simulink model "personal_transporter_model2_with_nonidealities"  (R2017a)
settings: Solver=VariableStepAuto  StartTime=0.0  StopTime=final_time  FixedStep=Ts  MaxStep=1  RelTol=1e-2
values from neighbouring files (symbols this model uses):
  alpha_c = 0.999    [digital_filters.m]
  beta_c = 1-alpha_c    (= 0.001)    [digital_filters.m]
  C_2 = [c11_2    0       -c11_2    0;      0      c11_2     -c11_2    0;      -c11_2   -c11_2    c33_2     c34_2;      0      0       c34_2     -c34_2]    [overall_model_2.m]
  D = 0.4    [param_personal_transporter_2_backup.m]    (also in vehicle_params.m = 0.5)
  Dec_2 = inv([1 1 0;0 0 1; 1 -1 0])    [overall_model_2.m]
  g = 9.81    [param_personal_transporter_2_backup.m]    (also in vehicle_params.m)
  iMAX = 2*iNom    (= 40)    [vehicle_params.m]
  k_PLL = 15    [digital_filters.m]
  k_s = 1440    [param_personal_transporter_2_backup.m]    (also in vehicle_params.m = 850)
  K_steer = dlqr(A_td,B_td,Q_steer,R_steer)    [steering_model_and_controller.m]
  Kd = dlqr(Ad,Bd,Q,R)    [equilibrium_model_and_controller.m]
  kt = ke    (= 0.0353677651315)    [param_personal_transporter_2_backup.m]    (also in vehicle_params.m = 0.694)
  L = P*C'*inv(C*P*C'+R)    [f_updating.m]    (also in f_updating_e.m; param_personal_transporter_2_backup.m = 0.9; vehicle_params.m = 0.1)
  m_P = 80    [param_personal_transporter_2_backup.m]    (also in vehicle_params.m = 30)
  n_hall = 3    [vehicle_params.m]
  r = 0.1    [param_personal_transporter_2_backup.m]    (also in vehicle_params.m)
  R_kalman_IMU = 20    [digital_filters.m]
  references_dot_delta = [  0 ,0;                         20, 0;                         23, 1;                         26, -1;                         29, 0;                         final_time, 0]    [steering_model_and_controller.m]
  references_dot_Xb = [ 0, 0;                     2.5, 0.5;                     5, 0;                     final_time, 0]    [equilibrium_model_and_controller.m]
  S = [ r/2  r/2  0;       r/D  -r/D 0;       0     0   1]    [overall_model.m]    (also in param_personal_transporter_2_backup.m = [ r/2  r/2  0  0;       r/D  -r/D 0  0;       0     0   1  0)
  S_2 = [ r/2  r/2  0  0;       r/D  -r/D 0  0;       0     0   1  0;       0     0   0  1]    [overall_model_2.m]
  Smot = [ rho  0   1;        0   rho  1;        0    0   1]    [overall_model.m]
  tacho_to_angle = (2*pi)/(n_poles*n_hall)    [vehicle_params.m]
  tau_PLL = omega_PLL    (= 31.4159265359)    [digital_filters.m]
  Ts = 0.01    [angle_fusion_readings.m]    (also in imu_model.m; other_stuff.m; param_personal_transporter.m; param_personal_transporter_2.m)
  U_2 = [1/rho 0 0;0 1/rho 0; -1/rho -1/rho -1; 0 0 1]    [overall_model_2.m]
undefined symbols (not defined in the file or in its folder): denF, denIloop, denIMU, denIMUint, denPI, denTorques, Discrete, n_poles, numF, numIloop, numIMU, numIMUint, numPI, numTorques, Time
libraries: simulink x5, ctrlSharedLib x2, cstblocks x1
settings Model: Creator=Dino Spiller  LastModifiedBy=mac_daino
settings SolverCC: ZeroCrossControl=DisableAll  InsertRTBMode=Never (minimum delay)
settings DataIOCC: LimitDataPoints=on  SaveFormat=Array  SignalLoggingSaveFormat=ModelDataLogs
settings OptimizationCC: ExpressionDepthLimit=2147483647  LifeSpan=inf
settings DebuggingCC: UnderspecifiedInitializationDetection=Classic  MergeDetectMultiDrivingBlocksExec=none  SolverPrmCheckMsg=warning  FcnCallInpInsideContextMsg=warning  StateNameClashWarn=warning  SFUnexpectedBacktrackingDiag=warning  SFNoUnconditionalDefaultTransitionDiag=warning  SFExecutionAtInitializationDiag=none
settings HardwareCC: ProdBitPerPointer=32  ProdBitPerSizeT=32  ProdBitPerPtrDiffT=32  ProdLargestAtomicFloat=None  ProdIntDivRoundTo=Undefined  ProdEndianess=Unspecified  ProdWordSize=32  ProdHWDeviceType=32-bit Generic
settings ModelReferenceCC: ModelReferenceMinAlgLoopOccurrences=on  PropagateSignalLabelsOutOfModel=off
settings RTWCC: CheckMdlBeforeBuild=Warning
settings GRTTargetCC: TargetLangStandard=C89/C90 (ANSI)  GeneratePreprocessorConditionals=Disable all  CombineOutputUpdateFcns=off  GRTInterface=on
settings ConfigComp: CovMetricSettings=dw  CovHtmlReporting=on  CovSaveCumulativeToWorkspaceVar=on  CovSaveSingleToWorkspaceVar=on  CovExternalEMLEnable=off

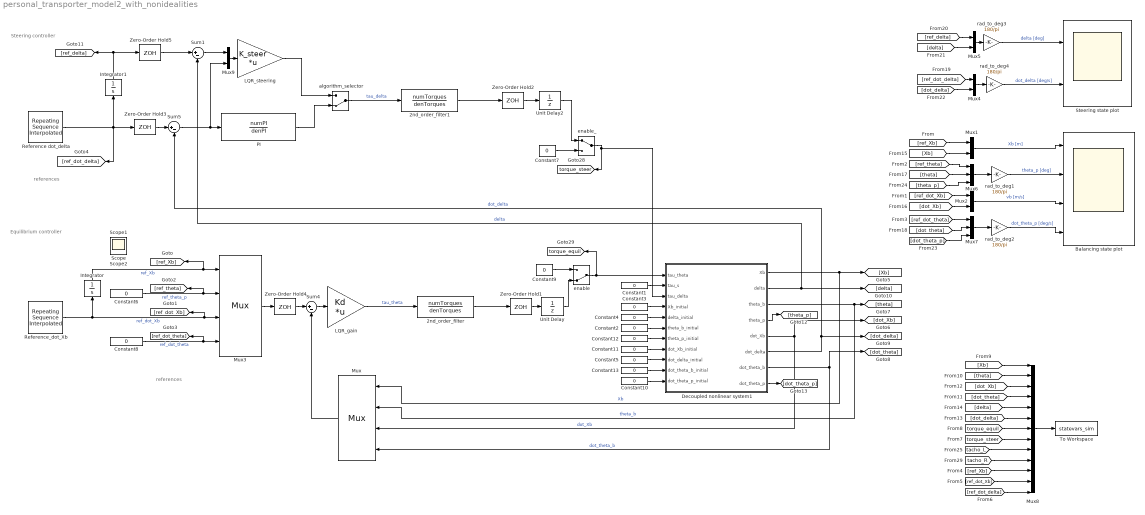
== system personal_transporter_model2_with_nonidealities ==
  note: Steering controller
  note: references
  note: Equilibrium controller
  note: references
  2nd_order_filter : DiscreteTransferFcn  Numerator=numTorques  Denominator=denTorques
  2nd_order_filter1 : DiscreteTransferFcn  Numerator=numTorques  Denominator=denTorques
  Balancing state plot : Scope  NumInputPorts=4
  Constant{1..13} (13 alike) : Constant  Value=0
  Decoupled nonlinear system1 : Subsystem
  Integrator : Integrator
  Integrator1 : Integrator
  LQR_gain : Gain  Gain=Kd  Multiplication=Matrix(K*u)
  LQR_steering : Gain  Gain=K_steer  Multiplication=Matrix(K*u)
  Mux : Mux
      settings: DisplayOption=signals
  Mux{1..2,4..5,9} (5 alike) : Mux  Inputs=2
  Mux3 : Mux
      settings: DisplayOption=signals
  Mux6 : Mux  Inputs=3
  Mux7 : Mux  Inputs=3
  Mux8 : Mux  Inputs=13
  PI : DiscreteTransferFcn  Numerator=numPI  Denominator=denPI
  Reference dot_delta : simulink/Sources/Repeating Sequence Interpolated  OutValues=references_dot_delta(:,2)  TimeValues=references_dot_delta(:,1)  LookUpMeth=Interpolation-Use End Values  tsamp=Ts  OutMin=[]  OutMax=[]  OutDataTypeStr=double  OutputDataTypeScalingMode=double  OutDataType=fixdt(0,8)  OutScaling=2^-10
  Reference_dot_Xb : simulink/Sources/Repeating Sequence Interpolated  OutValues=references_dot_Xb(:,2)  TimeValues=references_dot_Xb(:,1)  LookUpMeth=Interpolation-Use End Values  tsamp=Ts  OutMin=[]  OutMax=[]  OutDataTypeStr=double  OutputDataTypeScalingMode=double  OutDataType=fixdt(0,8)  OutScaling=2^-10
  Steering state plot : Scope  NumInputPorts=2
  Sum1 : Sum  Inputs=|+-
  Sum4 : Sum  Inputs=|+-
  Sum5 : Sum  Inputs=|+-
  To Workspace : ToWorkspace  VariableName=statevars_sim  SaveFormat=Timeseries  SampleTime=Ts
  Unit Delay : UnitDelay  SampleTime=Ts
  Unit Delay2 : UnitDelay  SampleTime=Ts
  Zero-Order Hold{1..5} (5 alike) : ZeroOrderHold  SampleTime=Ts
  algorithm_selector : ManualSwitch  CurrentSetting=0
  enable : ManualSwitch  CurrentSetting=0
  enable_ : ManualSwitch
  rad_to_deg{1..4} (4 alike) : Gain  Gain=180/pi
  Scope : Scope
  Scope1 : Scope
  Scope2 : Scope
  tag scope: torque_equil=global, torque_steer=global
  wires:
  Reference_dot_Xb/1 -> [ref_dot_Xb], Mux3/3, Integrator/1  "ref_dot_Xb"
  Decoupled nonlinear system1/1(Xb) -> [Xb], Mux/1  "Xb"
  Decoupled nonlinear system1/3(theta_b) -> [theta], Mux/2  "theta_b"
  Decoupled nonlinear system1/2(delta) -> Sum1/2, [delta]  "delta"
  Decoupled nonlinear system1/6(dot_delta) -> Sum5/2, [dot_delta]  "dot_delta"
  Constant3/1 -> Decoupled nonlinear system1/4(Xb_initial)
  Constant4/1 -> Decoupled nonlinear system1/5(delta_initial)
  Constant11/1 -> Decoupled nonlinear system1/8(dot_Xb_initial)
  Constant5/1 -> Decoupled nonlinear system1/9(dot_delta_initial)
  Constant10/1 -> Decoupled nonlinear system1/11(dot_theta_p_initial)
  enable/1 -> [torque_equil], Decoupled nonlinear system1/1("tau_theta ")
  Constant6/1 -> [ref_theta], Mux3/2  "ref_theta_p"
  Reference dot_delta/1 -> [ref_dot_delta], Zero-Order Hold3/1, Integrator1/1
  Constant7/1 -> enable_/2
  Zero-Order Hold2/1 -> Unit Delay2/1
  Mux4/1 -> rad_to_deg4/1
  Mux5/1 -> rad_to_deg3/1
  Integrator/1 -> [ref_Xb], Mux3/1  "ref_Xb"
  Constant8/1 -> [ref_dot_theta], Mux3/4  "ref_dot_theta"
  Mux3/1 -> Zero-Order Hold4/1
  Sum4/1 -> LQR_gain/1
  Mux/1 -> Sum4/2
  Sum5/1 -> Mux9/2, PI/1
  Mux1/1 -> Balancing state plot/1  "Xb [m]"
  [ref_Xb] -> Mux1/1
  [ref_dot_Xb] -> Mux2/1
  Zero-Order Hold4/1 -> Sum4/1
  Zero-Order Hold1/1 -> Unit Delay/1
  Mux8/1 -> To Workspace/1
  [torque_steer] -> Mux8/8
  [torque_equil] -> Mux8/7
  [tacho_L] -> Mux8/9
  [tacho_R] -> Mux8/10
  [ref_Xb] -> Mux8/11
  [ref_dot_Xb] -> Mux8/12
  [ref_dot_delta] -> Mux8/13
  Constant9/1 -> enable/1
  Unit Delay/1 -> enable/2
  [Xb] -> Mux8/1
  [theta] -> Mux8/2
  [dot_Xb] -> Mux8/3
  [dot_theta] -> Mux8/4
  [dot_delta] -> Mux8/6
  [delta] -> Mux8/5
  [Xb] -> Mux1/2
  [dot_Xb] -> Mux2/2
  Mux6/1 -> rad_to_deg1/1
  Mux2/1 -> Balancing state plot/3  "vb [m/s]"
  rad_to_deg1/1 -> Balancing state plot/2  "theta_p [deg]"
  [ref_theta] -> Mux6/1
  [theta] -> Mux6/2
  [ref_dot_theta] -> Mux7/1
  [dot_theta] -> Mux7/2
  Mux7/1 -> rad_to_deg2/1
  rad_to_deg2/1 -> Balancing state plot/4  "dot_theta_p [deg/s]"
  Unit Delay2/1 -> enable_/1
  Integrator1/1 -> Zero-Order Hold5/1, [ref_delta]
  rad_to_deg3/1 -> Steering state plot/1  "delta [deg]"
  rad_to_deg4/1 -> Steering state plot/2  "dot_delta [deg/s]"
  Zero-Order Hold3/1 -> Sum5/1
  Sum1/1 -> Mux9/1
  Mux9/1 -> LQR_steering/1
  LQR_steering/1 -> algorithm_selector/1
  PI/1 -> algorithm_selector/2
  algorithm_selector/1 -> 2nd_order_filter1/1  "tau_delta"
  [dot_delta] -> Mux4/2
  [ref_dot_delta] -> Mux4/1
  [delta] -> Mux5/2
  [ref_delta] -> Mux5/1
  Zero-Order Hold5/1 -> Sum1/1
  LQR_gain/1 -> 2nd_order_filter/1  "tau_theta"
  2nd_order_filter/1 -> Zero-Order Hold1/1
  enable_/1 -> Decoupled nonlinear system1/3(tau_delta), [torque_steer]
  2nd_order_filter1/1 -> Zero-Order Hold2/1
  Constant1/1 -> Decoupled nonlinear system1/2(tau_s)
  Constant2/1 -> Decoupled nonlinear system1/6(theta_b_initial)
  Constant12/1 -> Decoupled nonlinear system1/7(theta_p_initial)
  Constant13/1 -> Decoupled nonlinear system1/10(dot_theta_b_initial)
  Decoupled nonlinear system1/5("dot_Xb ") -> Mux/3, [dot_Xb]  "dot_Xb"
  Decoupled nonlinear system1/7(dot_theta_b) -> Mux/4, [dot_theta]  "dot_theta_b"
  Decoupled nonlinear system1/4(theta_p) -> [theta_p]
  Decoupled nonlinear system1/8(dot_theta_p) -> [dot_theta_p]
  [theta_p] -> Mux6/3
  [dot_theta_p] -> Mux7/3

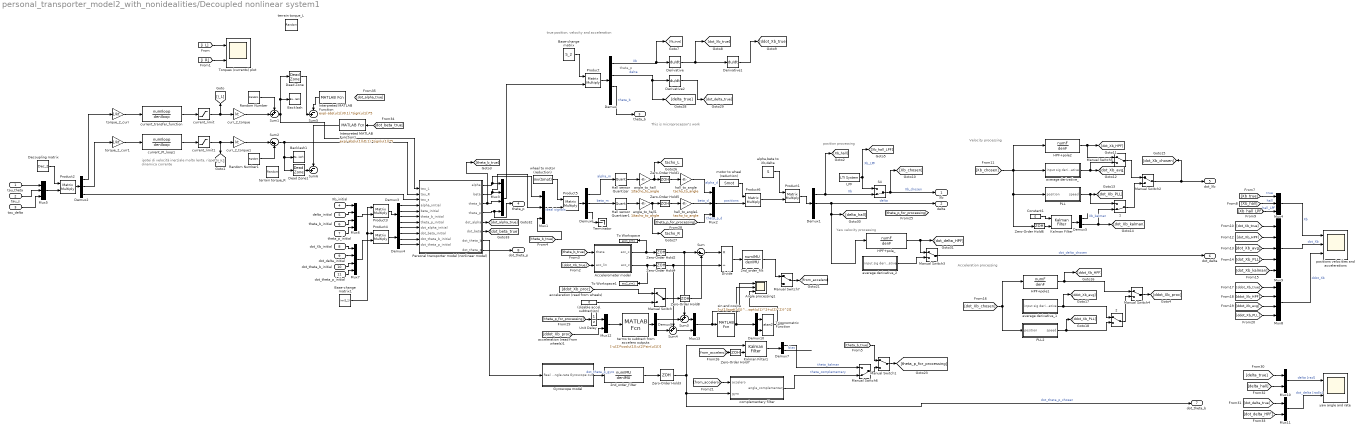
== system personal_transporter_model2_with_nonidealities/Decoupled nonlinear system1 ==
  note: theta_p
  note: ipotei di velocità  inerziale molto lenta, rispetto
      | a dinamica corrente
  note: Velocity processing
  note: Acceleration processing
  note: true position, velocity and acceleration
  note: position processing
  note: Yaw velocity processing
  note: This is microprocessor's work
  "tau_theta " : Inport
  tau_s : Inport  Port=2
  tau_delta : Inport  Port=3
  Xb_initial : Inport  Port=4
  delta_initial : Inport  Port=5
  theta_b_initial : Inport  Port=6
  theta_p_initial : Inport  Port=7
  dot_Xb_initial : Inport  Port=8
  dot_delta_initial : Inport  Port=9
  dot_theta_b_initial : Inport  Port=10
  dot_theta_p_initial : Inport  Port=11
  (disable accel. subtraction) : Constant  Value=0
  1 : ManualSwitch  CurrentSetting=0
  2 : ManualSwitch
  2nd_order_filt : DiscreteTransferFcn  Numerator=numIMU  Denominator=denIMU
  2nd_order_filter : DiscreteTransferFcn  Numerator=numIMU  Denominator=denIMU
  Accelerometer model : Subsystem
  Angle processing1 : Scope  NumInputPorts=3
  Backlash : Backlash  BacklashWidth=1.8
  Backlash1 : Backlash
  Base-change matrix : Constant  Value=S_2  VectorParams1D=off
  Base-change matrix1 : Constant  Value=inv(S_2)  VectorParams1D=off
  Constant1 : Constant  Value=0
  Dead Zone : DeadZone  LowerValue=-2  UpperValue=2  SaturateOnIntegerOverflow=on
  Dead Zone1 : DeadZone  LowerValue=-2  UpperValue=2  SaturateOnIntegerOverflow=on
  Decoupling matrix : Constant  Value=Dec_2  VectorParams1D=off
  Demux : Demux
  Demux1 : Demux  Outputs=3
  Demux{5,7,9..10} (4 alike) : Demux  Outputs=2
  Demux2 : Demux  Outputs=3
  Demux3 : Demux
  Demux4 : Demux
  Demux6 : Demux  Outputs=3
  Derivative : Derivative
  Derivative1 : Derivative
  Derivative2 : Derivative
  Divide : Product  Inputs=*/
  Gyroscope model : Subsystem
  HPF+pole1 : DiscreteTransferFcn  Numerator=numF  Denominator=denF  SampleTime=Ts
  HPF+pole2 : DiscreteTransferFcn  Numerator=numF  Denominator=denF  SampleTime=Ts
  HPF+pole_ : DiscreteTransferFcn  Numerator=numF  Denominator=denF
  Hall sensor Quantizer : Quantizer  QuantizationInterval=(2*pi)/(n_poles*n_hall)
  Hall sensor Quantizer1 : Quantizer  QuantizationInterval=(2*pi)/(n_poles*n_hall)
  Interpreted MATLAB Function : MATLABFcn  MATLABFcn=exp(-abs(u(1))/0.1).*sign(u(1))*5  OutputDimensions=[1]
  Interpreted MATLAB Function1 : MATLABFcn  MATLABFcn=exp(-abs(u(1))/0.1).*sign(u(1))*5  OutputDimensions=[1]
  Kalman Filter : ctrlSharedLib/Kalman Filter  TimeDomain=Discrete-Time  UseCurrentEstimator=on  ModelSource=Individual A, B, C, D matrices  ModelSourceVariable=ss(0.95,1,1,0,1)  A=[1 Ts; 0 1]  B=[0 ; 0]  C=[1 0]  D=0  NumberOfStates=1  NumberOfInputs=1  NumberOfOutputs=1  InitialEstimateSource=Dialog  X0=0  P0=10  UseK=off  UseGH=off  NumberOfProcessNoiseInputs=1  G=1  TimeInvariantG=on  H=0  TimeInvariantH=on  Q=[ 0.0001 0; 0 0.1]  TimeInvariantQ=on  R=4.06e-3  TimeInvariantR=on  N=0  TimeInvariantN=on  AddInputPort=on  AddEnablePort=off  OutputEstimatedY=off  OutputP=off  Ts=-1
  Kalman Filter1 : ctrlSharedLib/Kalman Filter  TimeDomain=Discrete-Time  UseCurrentEstimator=on  ModelSource=Individual A, B, C, D matrices  ModelSourceVariable=ss(0.95,1,1,0,1)  A=[1 -Ts; 0 1]  B=[Ts ; 0]  C=[1 0]  D=0  NumberOfStates=1  NumberOfInputs=1  NumberOfOutputs=1  InitialEstimateSource=Dialog  X0=0  P0=10  UseK=off  UseGH=off  NumberOfProcessNoiseInputs=1  G=1  TimeInvariantG=on  H=0  TimeInvariantH=on  Q=Q_kalman_IMU  TimeInvariantQ=on  R=R_kalman_IMU  TimeInvariantR=on  N=0  TimeInvariantN=on  AddInputPort=on  AddEnablePort=off  OutputEstimatedY=off  OutputP=off  Ts=-1
  LPF : cstblocks/LTI System  sys=LPF_c  IC=[]
  Manual Switch{,1..5,7} (7 alike) : ManualSwitch
  Manual Switch6 : ManualSwitch  CurrentSetting=0
  Mux{1..2,4..5} (4 alike) : Mux  Inputs=3
  Mux{10..13} (4 alike) : Mux  Inputs=2
  Mux{3,6..8} (4 alike) : Mux
  Mux9 : Mux  Inputs=5
  PLL : Subsystem
  PLL2 : Subsystem
  Personal transporter model (nonlinear model) : Subsystem
  Product{,1..6} (7 alike) : Product  Multiplication=Matrix(*)  RndMeth=Zero
  Random Number : RandomNumber  Variance=0.1  SampleTime=Ts
  Random Number1 : RandomNumber  Variance=0.1  Seed=50  SampleTime=Ts
  S4 : ManualSwitch  CurrentSetting=0
  Sum : Sum  Inputs=|+-
  Sum1 : Sum  Inputs=++|
  Sum2 : Sum  Inputs=|++
  Sum3 : Sum  Inputs=++|
  Sum4 : Sum  Inputs=++|
  Sum5 : Sum  Inputs=-+|
  Sum6 : Sum  Inputs=-+|
  Terminator : Terminator
  To Workspace : ToWorkspace  VariableName=accX_sim1  SaveFormat=Timeseries  SampleTime=-1
  To Workspace1 : ToWorkspace  VariableName=accZ_sim1  SaveFormat=Timeseries  SampleTime=-1
  Torques (currents) plot : Scope  NumInputPorts=2
  Trigonometric Function : Trigonometry  Operator=atan2
  Unit Delay : UnitDelay  InitialCondition=0.001  SampleTime=-1
  Zero-Order Hold{1..8} (8 alike) : ZeroOrderHold  SampleTime=Ts
  alpha,beta to Xb,delta : Constant  Value=S  VectorParams1D=off
  angle_to_hall : Gain  Gain=1/tacho_to_angle
  angle_to_hall1 : Gain  Gain=1/tacho_to_angle
  average derivative_ : Subsystem
  average derivative_1 : Subsystem
  average derivative_2 : Subsystem
  complementary filter : Subsystem
  curr_2_torque : Gain  Gain=kt
  curr_2_torque1 : Gain  Gain=kt
  current_PI_loop1 : DiscreteTransferFcn  Numerator=numIloop  Denominator=denIloop
  current_limit : Saturate  UpperLimit=iMAX  LowerLimit=-iMAX  LinearizeAsGain=off
  current_limit1 : Saturate  UpperLimit=iMAX  LowerLimit=-iMAX  LinearizeAsGain=off
  current_transfer_function : DiscreteTransferFcn  Numerator=numIloop  Denominator=denIloop
  hall_to_angle : Gain  Gain=tacho_to_angle
  hall_to_angle1 : Gain  Gain=tacho_to_angle
  motor to wheel (reduction) : Constant  Value=Smot  VectorParams1D=off
  positions velocities and accelerations : Scope  NumInputPorts=3
  sin and cosine : MATLABFcn  MATLABFcn=[-u(1)/sqrt(u(1)^2+u(2)^2); sqrt(1-(u(1)/sqrt(u(1)^2+u(2)^2))^2)]  OutputDimensions=[2,1]  Output1D=off
  terms to subtract from accelero outputs : MATLABFcn  MATLABFcn=[-u(2)*cos(u(1));u(2)*sin(u(1))]  OutputDimensions=[2,1]  Output1D=off
  terrain torque_L : UniformRandomNumber  Minimum=-0.1  Maximum=0.1  SampleTime=Ts
  terrain torque_R : UniformRandomNumber  Minimum=-0.1  Maximum=0.1  Seed=100  SampleTime=Ts
  torque_2_curr : Gain  Gain=1/kt
  torque_2_curr1 : Gain  Gain=1/kt
  wheel to motor (reduction) : Constant  Value=inv(Smot)  VectorParams1D=off
  yaw angle and rate : Scope  NumInputPorts=2
  Xb : Outport
  delta : Outport  Port=2
  theta_b : Outport  Port=3
  theta_p : Outport  Port=4
  "dot_Xb " : Outport  Port=5
  dot_delta : Outport  Port=6
  dot_theta_b : Outport  Port=7
  dot_theta_p : Outport  Port=8
  tag scope: tacho_L=global, tacho_R=global
  wires:
  Base-change matrix1/1 -> Product3/1, Product4/1
  dot_delta_initial/1 -> Mux7/2
  Decoupling matrix/1 -> Product2/1
  Product4/1 -> Demux4/1
  Mux7/1 -> Product4/2
  Demux3/2 -> Personal transporter model (nonlinear model)/5(beta_initial)
  Product3/1 -> Demux3/1
  Demux3/1 -> Personal transporter model (nonlinear model)/4(alpha_initial)
  Mux5/1 -> Product2/2
  Base-change matrix/1 -> Product/1
  Demux4/2 -> Personal transporter model (nonlinear model)/9(dot_beta_initial)
  Xb_initial/1 -> Mux6/1
  Demux4/1 -> Personal transporter model (nonlinear model)/8(dot_alpha_initial)
  delta_initial/1 -> Mux6/2
  dot_Xb_initial/1 -> Mux7/1
  Mux6/1 -> Product3/2
  Mux3/1 -> Product/2
  Demux/1 -> [Xb_true], Derivative/1  "Xb"
  Product/1 -> Demux/1
  Product2/1 -> Demux2/1
  "tau_theta "/1 -> Mux5/1
  Demux/2 -> Derivative2/1, [delta_true]  "delta"
  Personal transporter model (nonlinear model)/3(theta_b) -> [theta_b_true], Mux3/3
  Personal transporter model (nonlinear model)/4(theta_p) -> theta_p/1, Mux3/4
  Demux/3 -> theta_b/1  "theta_b"
  Demux3/4 -> Personal transporter model (nonlinear model)/7(theta_p_initial)
  Demux3/3 -> Personal transporter model (nonlinear model)/6(theta_b_initial)
  Demux4/3 -> Personal transporter model (nonlinear model)/10(dot_theta_b_initial)
  Demux4/4 -> Personal transporter model (nonlinear model)/11(dot_theta_p_initial)
  theta_p_initial/1 -> Mux6/4
  theta_b_initial/1 -> Mux6/3
  dot_theta_b_initial/1 -> Mux7/3
  dot_theta_p_initial/1 -> Mux7/4
  tau_s/1 -> Mux5/2
  tau_delta/1 -> Mux5/3
  Demux2/3 -> Personal transporter model (nonlinear model)/3(tau_s)
  current_limit1/1 -> curr_2_torque1/1, [i_R]
  [i_L] -> Torques (currents) plot/1
  Demux2/1 -> torque_2_curr/1
  curr_2_torque/1 -> Sum1/2
  Demux2/2 -> torque_2_curr1/1
  Sum1/1 -> Personal transporter model (nonlinear model)/1("tau_L "), Dead Zone/1, Backlash/1
  curr_2_torque1/1 -> Sum2/1
  torque_2_curr/1 -> current_transfer_function/1
  [i_R] -> Torques (currents) plot/2
  current_limit/1 -> [i_L], curr_2_torque/1
  Sum2/1 -> Personal transporter model (nonlinear model)/2("tau_R "), Backlash1/1, Dead Zone1/1
  Interpreted MATLAB Function1/1 -> Sum6/1
  [dot_beta_true] -> Interpreted MATLAB Function1/1
  current_PI_loop1/1 -> current_limit1/1
  torque_2_curr1/1 -> current_PI_loop1/1
  Random Number1/1 -> Sum2/2
  Interpreted MATLAB Function/1 -> Sum5/1
  Random Number/1 -> Sum1/1
  Dead Zone1/1 -> Sum6/2
  Dead Zone/1 -> Sum5/2
  current_transfer_function/1 -> current_limit/1
  Demux10/1 -> Trigonometric Function/1
  Zero-Order Hold6/1 -> Kalman Filter/2
  Zero-Order Hold7/1 -> Kalman Filter1/2
  Demux6/2 -> Hall sensor Quantizer1/1  "beta_m"
  Personal transporter model (nonlinear model)/1(alpha) -> Mux1/1, Mux3/1
  Demux6/1 -> Hall sensor Quantizer/1  "alpha_m"
  [ddot_Xb_HPF] -> Mux8/2
  wheel to motor (reduction)/1 -> Product5/1
  [delta_true] -> Mux10/1
  Personal transporter model (nonlinear model)/7(dot_theta_b) -> Gyroscope model/1(Real angle-rate)
  average derivative_/1(derivative) -> [dot_Xb_avg], Manual Switch5/2
  [ddot_Xb_true] -> Accelerometer model/2(acc_lin)
  angle_to_hall1/1 -> Zero-Order Hold5/1, [tacho_R]
  Manual Switch2/1 -> "dot_Xb "/1, [dot_Xb_chosen]
  [delta_hall] -> Mux10/2
  Mux1/1 -> Product5/2  "ideal signals"
  Demux7/2 -> ?  "bias"
  PLL/1("speed ") -> [dot_Xb_PLL], 1/1
  [dot_Xb_avg] -> Mux9/3
  [dot_delta_true] -> Mux11/1
  Accelerometer model/2(acc_z) -> To Workspace1/1, Zero-Order Hold4/1
  sin and cosine/1 -> Demux10/1, Angle processing1/2
  hall_to_angle/1 -> Mux2/1  "alpha_d"
  angle_to_hall/1 -> [tacho_L], Zero-Order Hold1/1
  Product6/1 -> Product1/2
  Manual Switch3/1 -> dot_delta/1  "dot_delta_chosen"
  Mux11/1 -> yaw angle and rate/2  "dot_delta [rad/s]"
  (disable accel. subtraction)/1 -> Manual Switch/2
  Mux2/1 -> Product6/2  "positions"
  LPF/1 -> [Xb_hall_LPF], S4/1  "Xb_LPF"
  Personal transporter model (nonlinear model)/2(beta) -> Mux1/2, Mux3/2
  Manual Switch5/1 -> Manual Switch2/1
  alpha,beta to Xb,delta/1 -> Product1/1
  Manual Switch1/1 -> [theta_p_for_processing]
  Constant1/1 -> Kalman Filter/1
  [Xb_hall_LPF] -> Mux4/3  "hall_LPF"
  Demux1/2 -> delta/1, [delta_hall], HPF+pole_/1  "delta"
  Derivative1/1 -> [ddot_Xb_true]
  [dot_Xb_kalman] -> Mux9/5
  HPF+pole1/1 -> [ddot_Xb_HPF], Manual Switch4/1
  [theta_b_true] -> Accelerometer model/1(theta)
  Mux4/1 -> positions velocities and accelerations/1  "Xb"
  [dot_Xb_HPF] -> Mux9/2
  Demux9/1 -> Sum3/2
  Zero-Order Hold8/1 -> Sum/2
  Zero-Order Hold3/1 -> complementary filter/2(gyro), dot_theta_b/1, Kalman Filter1/1  "dot_theta_p_chosen"
  motor to wheel (reduction)/1 -> Product6/1
  [Xb_true] -> Mux4/1  "true"
  1/1 -> Manual Switch2/2
  Product1/1 -> Demux1/1
  2/1 -> Manual Switch4/2
  [Xb_hall] -> Mux4/2  "hall"
  Kalman Filter1/1 -> Demux7/1
  [dot_delta_HPF] -> Mux11/2
  [dot_Xb_chosen] -> PLL2/1(position), HPF+pole1/1
  Zero-Order Hold1/1 -> hall_to_angle/1
  Demux1/1 -> [Xb_hall], S4/2  "Xb"
  [from_accelero] -> Zero-Order Hold7/1
  Zero-Order Hold2/1 -> Sum3/1, Sum/1
  [ddot_Xb_proc] -> Mux12/2
  Demux7/1 -> Manual Switch6/1  "theta_kalman"
  [from_accelero] -> complementary filter/1(accelero)
  Manual Switch/1 -> Zero-Order Hold8/1
  [Xb_chosen] -> HPF+pole2/1, PLL/1(position), Zero-Order Hold6/1, average derivative_/1(input sig)
  Mux9/1 -> positions velocities and accelerations/2  "dot_Xb"
  S4/1 -> Xb/1, [Xb_chosen]  "Xb_chosen"
  [theta_b_true] -> Manual Switch1/1
  Manual Switch4/1 -> [ddot_Xb_proc]
  Hall sensor Quantizer1/1 -> angle_to_hall1/1
  Manual Switch7/1 -> [from_accelero]
  [theta_p_for_processing] -> Unit Delay/1
  Gyroscope model/1(Gyroscope out) -> 2nd_order_filter/1  "dot_theta_p_gyro"
  Zero-Order Hold4/1 -> Sum4/1, Divide/2
  Derivative2/1 -> [dot_delta_true]
  [theta_p_for_processing] -> Mux2/3  "theta_p_d"
  [ddot_Xb_PLL] -> Mux8/4
  [ddot_Xb_proc] -> Manual Switch/1
  Demux5/1 -> ?  "Xb_kalman"
  Mux12/1 -> terms to subtract from accelero outputs/1
  Derivative/1 -> [dot_Xb_true], Derivative1/1
  Zero-Order Hold5/1 -> hall_to_angle1/1
  Hall sensor Quantizer/1 -> angle_to_hall/1
  Trigonometric Function/1 -> Angle processing1/3
  Mux10/1 -> yaw angle and rate/1  "delta [rad]"
  Mux8/1 -> positions velocities and accelerations/3  "ddot_Xb"
  Manual Switch6/1 -> Manual Switch1/2
  2nd_order_filter/1 -> Zero-Order Hold3/1
  HPF+pole_/1 -> [dot_delta_HPF], Manual Switch3/1
  Kalman Filter/1 -> Demux5/1
  [ddot_Xb_true] -> Mux8/1
  average derivative_1/1(derivative) -> 2/1, [ddot_Xb_avg]
  [dot_Xb_true] -> Mux9/1
  Demux9/2 -> Sum4/2
  Mux13/1 -> Angle processing1/1, sin and cosine/1
  [ddot_Xb_avg] -> Mux8/3
  PLL2/1("speed ") -> [ddot_Xb_PLL], 2/2
  Sum/1 -> Divide/1
  Demux10/2 -> Trigonometric Function/2
  complementary filter/1(angle_complementary) -> Manual Switch6/2  "theta_complementary"
  terms to subtract from accelero outputs/1 -> Demux9/1
  HPF+pole2/1 -> Manual Switch5/1, [dot_Xb_HPF]
  [dot_Xb_PLL] -> Mux9/4
  Divide/1 -> 2nd_order_filt/1
  Product5/1 -> Demux6/1
  Sum3/1 -> Mux13/1
  Sum4/1 -> Mux13/2
  Demux5/2 -> [dot_Xb_kalman], 1/2
  average derivative_2/1(derivative) -> Manual Switch3/2
  Accelerometer model/1(acc_x) -> To Workspace/1, Zero-Order Hold2/1
  hall_to_angle1/1 -> Mux2/2  "beta_d"
  2nd_order_filt/1 -> Manual Switch7/1
  Unit Delay/1 -> Mux12/1
  Personal transporter model (nonlinear model)/5(dot_alpha) -> [dot_alpha_true]
  Personal transporter model (nonlinear model)/6(dot_beta) -> [dot_beta_true]
  Personal transporter model (nonlinear model)/8(dot_theta_p) -> dot_theta_p/1
  [theta_b_true] -> Mux1/3
  Demux6/3 -> Terminator/1

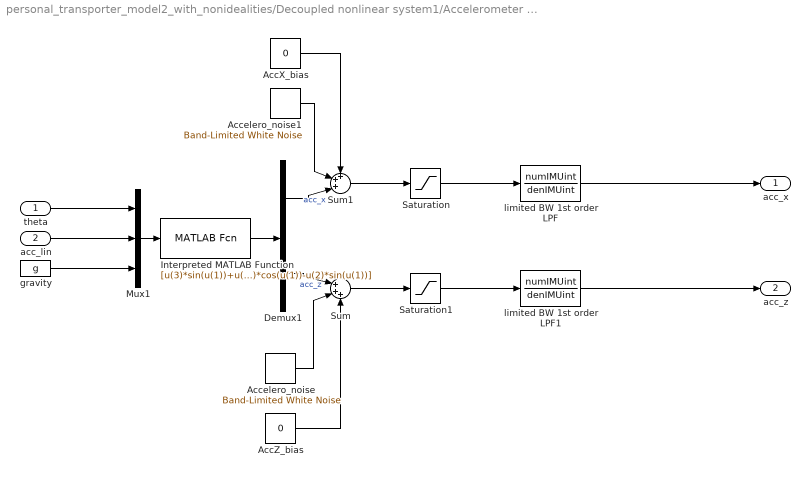
== system personal_transporter_model2_with_nonidealities/Decoupled nonlinear system1/Accelerometer model ==
  theta : Inport
  acc_lin : Inport  Port=2
  AccX_bias : Constant  Value=0
  AccZ_bias : Constant  Value=0
  Accelero_noise : simulink/Sources/Band-Limited White Noise  Cov=[((300*10^(-6))*g)^2]  Ts=Ts  seed=[23341]
  Accelero_noise1 : simulink/Sources/Band-Limited White Noise  Cov=[((300*10^(-6))*g)^2]  Ts=Ts  seed=[214321]
  Demux1 : Demux  Outputs=2
  Interpreted MATLAB Function : MATLABFcn  MATLABFcn=[u(3)*sin(u(1))+u(2)*cos(u(1));u(3)*cos(u(1))-u(2)*sin(u(1))]  OutputDimensions=[2,1]  Output1D=off
  Mux1 : Mux  Inputs=3
  Saturation : Saturate  UpperLimit=2*g  LowerLimit=-2*g
  Saturation1 : Saturate  UpperLimit=2*g  LowerLimit=-2*g
  Sum : Sum  Inputs=|+++
  Sum1 : Sum  Inputs=+++|
  gravity : Constant  Value=g
  limited BW 1st order LPF : DiscreteTransferFcn  Numerator=numIMUint  Denominator=denIMUint  SampleTime=Ts
  limited BW 1st order LPF1 : DiscreteTransferFcn  Numerator=numIMUint  Denominator=denIMUint  InitialStates=g  SampleTime=Ts
  acc_x : Outport
  acc_z : Outport  Port=2
  wires:
  Mux1/1 -> Interpreted MATLAB Function/1
  Interpreted MATLAB Function/1 -> Demux1/1
  gravity/1 -> Mux1/3
  Demux1/2 -> Sum/1  "acc_z"
  acc_lin/1 -> Mux1/2
  theta/1 -> Mux1/1
  Accelero_noise/1 -> Sum/2
  Saturation/1 -> limited BW 1st order LPF/1
  Saturation1/1 -> limited BW 1st order LPF1/1
  Demux1/1 -> Sum1/3  "acc_x"
  Accelero_noise1/1 -> Sum1/2
  Sum1/1 -> Saturation/1
  Sum/1 -> Saturation1/1
  limited BW 1st order LPF/1 -> acc_x/1
  limited BW 1st order LPF1/1 -> acc_z/1
  AccZ_bias/1 -> Sum/3
  AccX_bias/1 -> Sum1/1

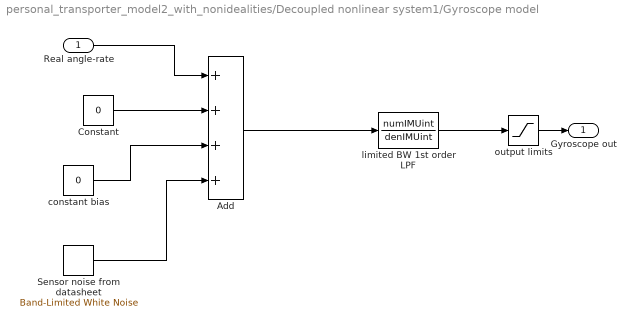
== system personal_transporter_model2_with_nonidealities/Decoupled nonlinear system1/Gyroscope model ==
  Real angle-rate : Inport
  Add : Sum  Inputs=++++
  Constant : Constant  Value=0
  "Sensor noise from datasheet " : simulink/Sources/Band-Limited White Noise  Cov=[(0.01*2*pi/180)^2]  Ts=Ts  seed=[24341]
  constant bias : Constant  Value=0
  limited BW 1st order LPF : DiscreteTransferFcn  Numerator=numIMUint  Denominator=denIMUint
  output limits : Saturate  UpperLimit=250*2*pi/180  LowerLimit=-250*2*pi/180
  Gyroscope out : Outport
  wires:
  limited BW 1st order LPF/1 -> output limits/1
  output limits/1 -> Gyroscope out/1
  "Sensor noise from datasheet "/1 -> Add/4
  Real angle-rate/1 -> Add/1
  Add/1 -> limited BW 1st order LPF/1
  constant bias/1 -> Add/3
  Constant/1 -> Add/2

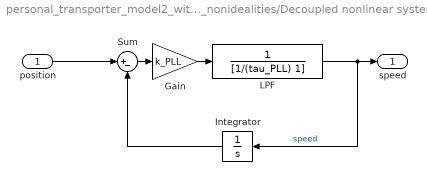
== system personal_transporter_model2_with_nonidealities/Decoupled nonlinear system1/PLL ==
  position : Inport
  Gain : Gain  Gain=k_PLL
  Integrator : Integrator
  LPF : TransferFcn  Denominator=[1/(tau_PLL) 1]
  Sum : Sum  Inputs=|+-
  "speed " : Outport
  wires:
  position/1 -> Sum/1
  Sum/1 -> Gain/1
  Integrator/1 -> Sum/2
  Gain/1 -> LPF/1
  LPF/1 -> "speed "/1, Integrator/1  "speed"

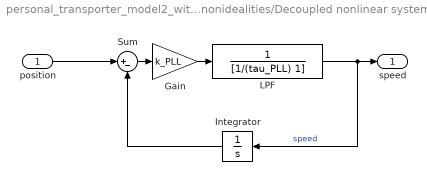
== system personal_transporter_model2_with_nonidealities/Decoupled nonlinear system1/PLL2 ==
  position : Inport
  Gain : Gain  Gain=k_PLL
  Integrator : Integrator
  LPF : TransferFcn  Denominator=[1/(tau_PLL) 1]
  Sum : Sum  Inputs=|+-
  "speed " : Outport
  wires:
  position/1 -> Sum/1
  Sum/1 -> Gain/1
  Integrator/1 -> Sum/2
  Gain/1 -> LPF/1
  LPF/1 -> "speed "/1, Integrator/1  "speed"

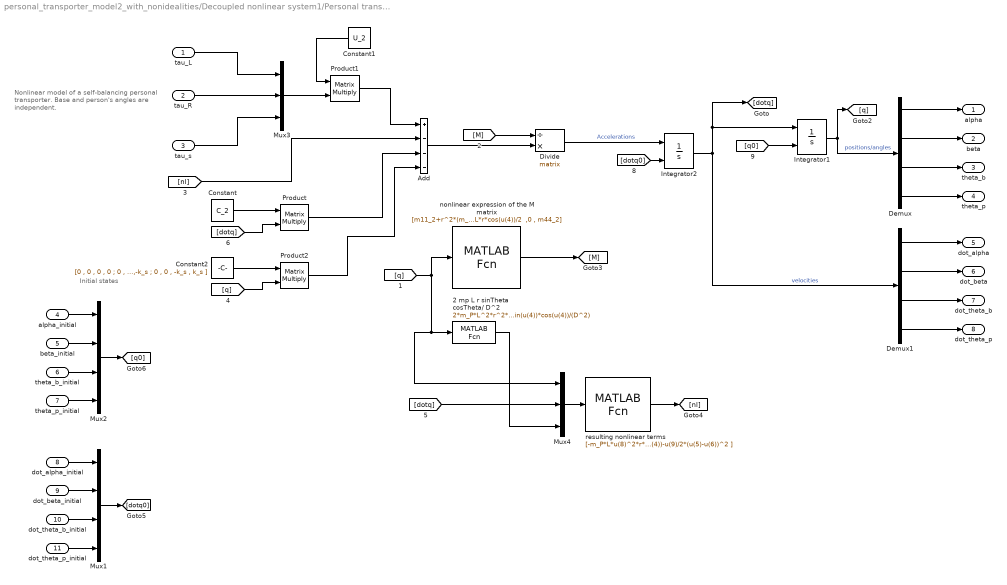
== system personal_transporter_model2_with_nonidealities/Decoupled nonlinear system1/Personal transporter model (nonlinear model) ==
  note: Initial states
  note: Nonlinear model of a self-balancing
      | personal transporter.
      | Base and person's angles are independent.
  "tau_L " : Inport
  "tau_R " : Inport  Port=2
  tau_s : Inport  Port=3
  alpha_initial : Inport  Port=4
  beta_initial : Inport  Port=5
  theta_b_initial : Inport  Port=6
  theta_p_initial : Inport  Port=7
  dot_alpha_initial : Inport  Port=8
  dot_beta_initial : Inport  Port=9
  dot_theta_b_initial : Inport  Port=10
  dot_theta_p_initial : Inport  Port=11
  2 mp L r sinTheta cosTheta/ D^2 : MATLABFcn  MATLABFcn=2*m_P*L^2*r^2*sin(u(4))*cos(u(4))/(D^2)  OutputDimensions=[1]  Output1D=off
  Add : Sum  Inputs=+---
  Constant : Constant  Value=C_2  VectorParams1D=off
  Constant1 : Constant  Value=U_2  VectorParams1D=off
  Constant2 : Constant  Value=[0 , 0 , 0 , 0 ; 0 , 0 , 0 , 0 ; 0 , 0 , k_s ,-k_s ; 0 , 0 , -k_s , k_s ]  VectorParams1D=off
  Demux : Demux
  Demux1 : Demux
  Divide : Product  Inputs=/*  Multiplication=Matrix(*)
  Integrator1 : Integrator  InitialConditionSource=external  InitialCondition=[0; 5*pi/180]
  Integrator2 : Integrator  InitialConditionSource=external  InitialCondition=[0; 5*pi/180]
  Mux1 : Mux
  Mux2 : Mux
  Mux3 : Mux  Inputs=3
  Mux4 : Mux  Inputs=3
  Product : Product  Multiplication=Matrix(*)  RndMeth=Zero
  Product1 : Product  Multiplication=Matrix(*)  RndMeth=Zero
  Product2 : Product  Multiplication=Matrix(*)  RndMeth=Zero
  nonlinear expression of the M matrix : MATLABFcn  MATLABFcn="[m11_2+r^2*(m_P*L^2*sin(u(4))^2)/D^2  ,  m12_2-r^2*(m_P*L^2*sin(u(4))^2)/D^2  ,  m13_2  ,  m_P*L*r*cos(u(4))/2  ; m12_2-r^2*(m_P*L^2*sin(u(3))^2)/D^2  ,  m11_2+r^2*(m_P*L^2*sin(u(3))^2)/D^2  ,  m13_2  ,  m_P*L*r*cos(u(4))/2  ; m13_2  ,  m13_2  ,  m33_2  ,  0  ; m_P*L*r*cos(u(4))/2  ,  m_P*L*r*cos(u(4))/2  ,0 , m44_2]"  OutputDimensions=[4,4]  Output1D=off
  resulting nonlinear terms : MATLABFcn  MATLABFcn="[-m_P*L*u(8)^2*r*sin(u(4))/2+u(9)*u(8)*(u(5)-u(6)) ;  -m_P*L*u(8)^2*r*sin(u(4))/2+u(9)*u(8)*(u(6)-u(5))  ;  0   ;  -m_P*g*L*sin(u(4))-u(9)/2*(u(5)-u(6))^2 ]"  OutputDimensions=[4,1]  Output1D=off
  alpha : Outport
  beta : Outport  Port=2
  theta_b : Outport  Port=3
  theta_p : Outport  Port=4
  dot_alpha : Outport  Port=5
  dot_beta : Outport  Port=6
  dot_theta_b : Outport  Port=7
  dot_theta_p : Outport  Port=8
  wires:
  Integrator1/1 -> [q], Demux/1  "positions/angles"
  Integrator2/1 -> [dotq], Integrator1/1, Demux1/1  "velocities"
  Divide/1 -> Integrator2/1  "Accelerations"
  nonlinear expression of the M matrix/1 -> [M]
  [M] -> Divide/1
  Add/1 -> Divide/2
  Demux/1 -> alpha/1
  Demux/2 -> beta/1
  Product/1 -> Add/3
  alpha_initial/1 -> Mux2/1
  beta_initial/1 -> Mux2/2
  Mux2/1 -> [q0]
  [dotq0] -> Integrator2/2
  [q0] -> Integrator1/2
  Constant/1 -> Product/1
  2 mp L r sinTheta cosTheta/ D^2/1 -> Mux4/3
  [nl] -> Add/2
  Demux/3 -> theta_b/1
  Demux1/2 -> dot_beta/1
  Demux1/1 -> dot_alpha/1
  dot_beta_initial/1 -> Mux1/2
  dot_alpha_initial/1 -> Mux1/1
  Mux1/1 -> [dotq0]
  [q] -> Mux4/1, 2 mp L r sinTheta cosTheta/ D^2/1, nonlinear expression of the M matrix/1
  Product1/1 -> Add/1
  Constant1/1 -> Product1/1
  Mux3/1 -> Product1/2
  "tau_L "/1 -> Mux3/1
  "tau_R "/1 -> Mux3/2
  [dotq] -> Mux4/2
  [dotq] -> Product/2
  Mux4/1 -> resulting nonlinear terms/1
  resulting nonlinear terms/1 -> [nl]
  Demux/4 -> theta_p/1
  Demux1/3 -> dot_theta_b/1
  Demux1/4 -> dot_theta_p/1
  tau_s/1 -> Mux3/3
  theta_p_initial/1 -> Mux2/4
  theta_b_initial/1 -> Mux2/3
  dot_theta_p_initial/1 -> Mux1/4
  dot_theta_b_initial/1 -> Mux1/3
  [q] -> Product2/2
  Product2/1 -> Add/4
  Constant2/1 -> Product2/1

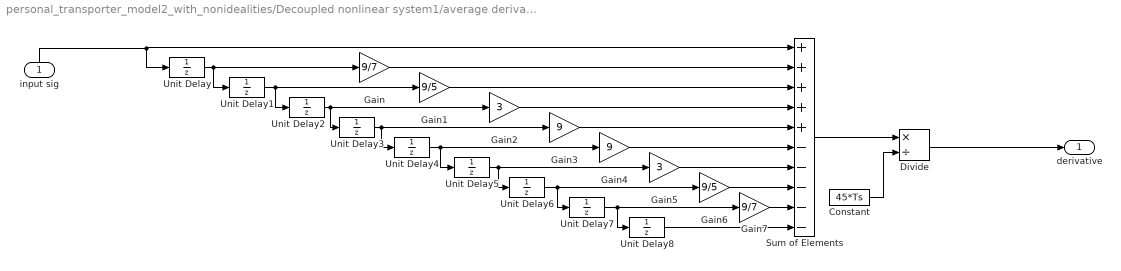
== system personal_transporter_model2_with_nonidealities/Decoupled nonlinear system1/average derivative_ ==
  input sig : Inport
  Constant : Constant  Value=45*Ts
  Divide : Product  Inputs=*/
  Gain : Gain  Gain=9/7
  Gain1 : Gain  Gain=9/5
  Gain2 : Gain  Gain=3
  Gain3 : Gain  Gain=9
  Gain4 : Gain  Gain=9
  Gain5 : Gain  Gain=3
  Gain6 : Gain  Gain=9/5
  Gain7 : Gain  Gain=9/7
  Sum of Elements : Sum  Inputs=+++++-----
  Unit Delay{,1..8} (9 alike) : UnitDelay  SampleTime=Ts
  derivative : Outport
  wires:
  input sig/1 -> Sum of Elements/1, Unit Delay/1
  Unit Delay/1 -> Gain/1, Unit Delay1/1
  Unit Delay8/1 -> Sum of Elements/10
  Unit Delay4/1 -> Gain4/1, Unit Delay5/1
  Unit Delay5/1 -> Gain5/1, Unit Delay6/1
  Unit Delay6/1 -> Unit Delay7/1, Gain6/1
  Unit Delay2/1 -> Gain2/1, Unit Delay3/1
  Unit Delay1/1 -> Gain1/1, Unit Delay2/1
  Unit Delay3/1 -> Gain3/1, Unit Delay4/1
  Unit Delay7/1 -> Gain7/1, Unit Delay8/1
  Divide/1 -> derivative/1
  Gain/1 -> Sum of Elements/2
  Gain1/1 -> Sum of Elements/3
  Gain2/1 -> Sum of Elements/4
  Gain3/1 -> Sum of Elements/5
  Gain7/1 -> Sum of Elements/9
  Sum of Elements/1 -> Divide/1
  Constant/1 -> Divide/2
  Gain6/1 -> Sum of Elements/8
  Gain5/1 -> Sum of Elements/7
  Gain4/1 -> Sum of Elements/6

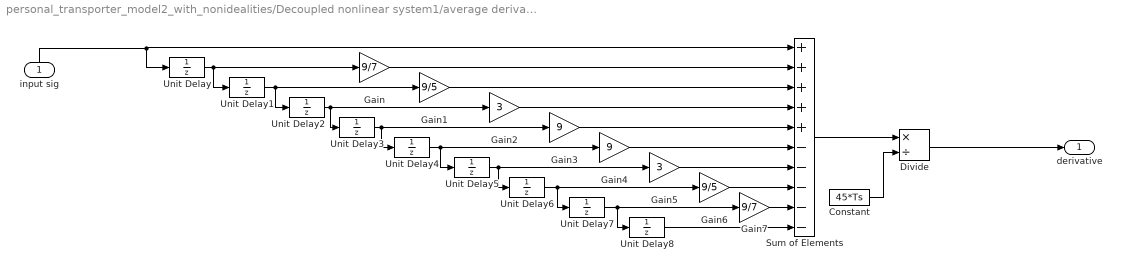
== system personal_transporter_model2_with_nonidealities/Decoupled nonlinear system1/average derivative_1 ==
  input sig : Inport
  Constant : Constant  Value=45*Ts
  Divide : Product  Inputs=*/
  Gain : Gain  Gain=9/7
  Gain1 : Gain  Gain=9/5
  Gain2 : Gain  Gain=3
  Gain3 : Gain  Gain=9
  Gain4 : Gain  Gain=9
  Gain5 : Gain  Gain=3
  Gain6 : Gain  Gain=9/5
  Gain7 : Gain  Gain=9/7
  Sum of Elements : Sum  Inputs=+++++-----
  Unit Delay{,1..8} (9 alike) : UnitDelay  SampleTime=Ts
  derivative : Outport
  wires:
  input sig/1 -> Sum of Elements/1, Unit Delay/1
  Unit Delay/1 -> Gain/1, Unit Delay1/1
  Unit Delay8/1 -> Sum of Elements/10
  Unit Delay4/1 -> Gain4/1, Unit Delay5/1
  Unit Delay5/1 -> Gain5/1, Unit Delay6/1
  Unit Delay6/1 -> Unit Delay7/1, Gain6/1
  Unit Delay2/1 -> Gain2/1, Unit Delay3/1
  Unit Delay1/1 -> Gain1/1, Unit Delay2/1
  Unit Delay3/1 -> Gain3/1, Unit Delay4/1
  Unit Delay7/1 -> Gain7/1, Unit Delay8/1
  Divide/1 -> derivative/1
  Gain/1 -> Sum of Elements/2
  Gain1/1 -> Sum of Elements/3
  Gain2/1 -> Sum of Elements/4
  Gain3/1 -> Sum of Elements/5
  Gain7/1 -> Sum of Elements/9
  Sum of Elements/1 -> Divide/1
  Constant/1 -> Divide/2
  Gain6/1 -> Sum of Elements/8
  Gain5/1 -> Sum of Elements/7
  Gain4/1 -> Sum of Elements/6

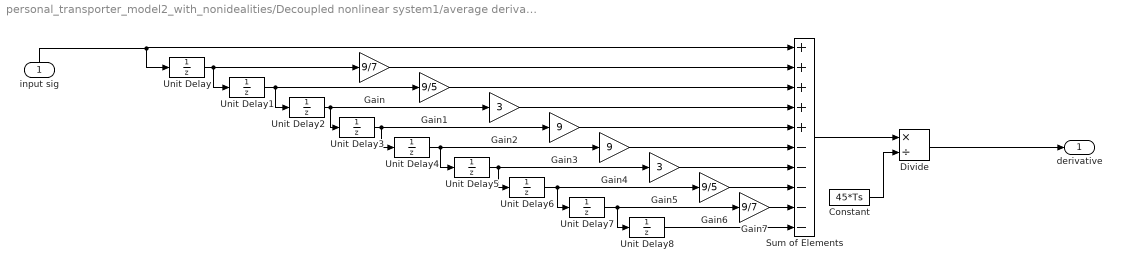
== system personal_transporter_model2_with_nonidealities/Decoupled nonlinear system1/average derivative_2 ==
  input sig : Inport
  Constant : Constant  Value=45*Ts
  Divide : Product  Inputs=*/
  Gain : Gain  Gain=9/7
  Gain1 : Gain  Gain=9/5
  Gain2 : Gain  Gain=3
  Gain3 : Gain  Gain=9
  Gain4 : Gain  Gain=9
  Gain5 : Gain  Gain=3
  Gain6 : Gain  Gain=9/5
  Gain7 : Gain  Gain=9/7
  Sum of Elements : Sum  Inputs=+++++-----
  Unit Delay{,1..8} (9 alike) : UnitDelay  SampleTime=Ts
  derivative : Outport
  wires:
  input sig/1 -> Sum of Elements/1, Unit Delay/1
  Unit Delay/1 -> Gain/1, Unit Delay1/1
  Unit Delay8/1 -> Sum of Elements/10
  Unit Delay4/1 -> Gain4/1, Unit Delay5/1
  Unit Delay5/1 -> Gain5/1, Unit Delay6/1
  Unit Delay6/1 -> Unit Delay7/1, Gain6/1
  Unit Delay2/1 -> Gain2/1, Unit Delay3/1
  Unit Delay1/1 -> Gain1/1, Unit Delay2/1
  Unit Delay3/1 -> Gain3/1, Unit Delay4/1
  Unit Delay7/1 -> Gain7/1, Unit Delay8/1
  Divide/1 -> derivative/1
  Gain/1 -> Sum of Elements/2
  Gain1/1 -> Sum of Elements/3
  Gain2/1 -> Sum of Elements/4
  Gain3/1 -> Sum of Elements/5
  Gain7/1 -> Sum of Elements/9
  Sum of Elements/1 -> Divide/1
  Constant/1 -> Divide/2
  Gain6/1 -> Sum of Elements/8
  Gain5/1 -> Sum of Elements/7
  Gain4/1 -> Sum of Elements/6

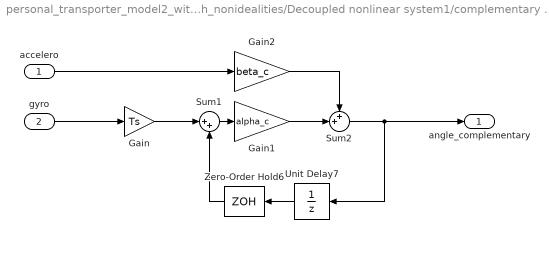
== system personal_transporter_model2_with_nonidealities/Decoupled nonlinear system1/complementary filter ==
  accelero : Inport
  gyro : Inport  Port=2
  Gain : Gain  Gain=Ts
  Gain1 : Gain  Gain=alpha_c
  Gain2 : Gain  Gain=beta_c
  Sum1 : Sum  Inputs=|++
  Sum2 : Sum  Inputs=++|
  Unit Delay7 : UnitDelay  SampleTime=Ts
  Zero-Order Hold6 : ZeroOrderHold  SampleTime=Ts
  angle_complementary : Outport
  wires:
  Gain1/1 -> Sum2/2
  Gain2/1 -> Sum2/1
  Zero-Order Hold6/1 -> Sum1/2
  Gain/1 -> Sum1/1
  Sum1/1 -> Gain1/1
  Sum2/1 -> Unit Delay7/1, angle_complementary/1
  accelero/1 -> Gain2/1
  gyro/1 -> Gain/1
  Unit Delay7/1 -> Zero-Order Hold6/1
